simulink model "update"  (R2024a)
settings: Solver=VariableStepAuto  StartTime=0.0  StopTime=10.0  RelTol=1e-3
values from neighbouring files (symbols this model uses):
  c = 0.004    [model_constants.m]
  g = 9.81    [model_constants.m]
  J = 10.183e-4    (= 0.0010183)    [model_constants.m]
  k = 0.1    [model_constants.m]
  ke = 0.083    [model_constants.m]
  ki = 0.004    [model_constants.m]
  L = 0.134    [model_constants.m]
  m = 43.4    [model_constants.m]
  R = 0.5    [model_constants.m]
  x = 2    [model_constants.m]
libraries: simulink x2
settings Model: PacingRate=0.280000  Creator=tinas  LastModifiedBy=tinas

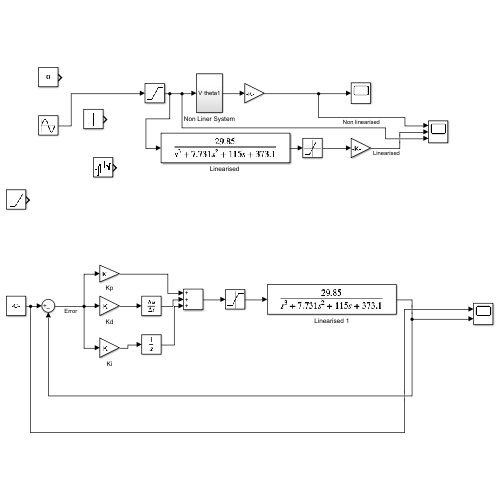
[thumbnail: Simulink's stored preview of the top-level diagram]
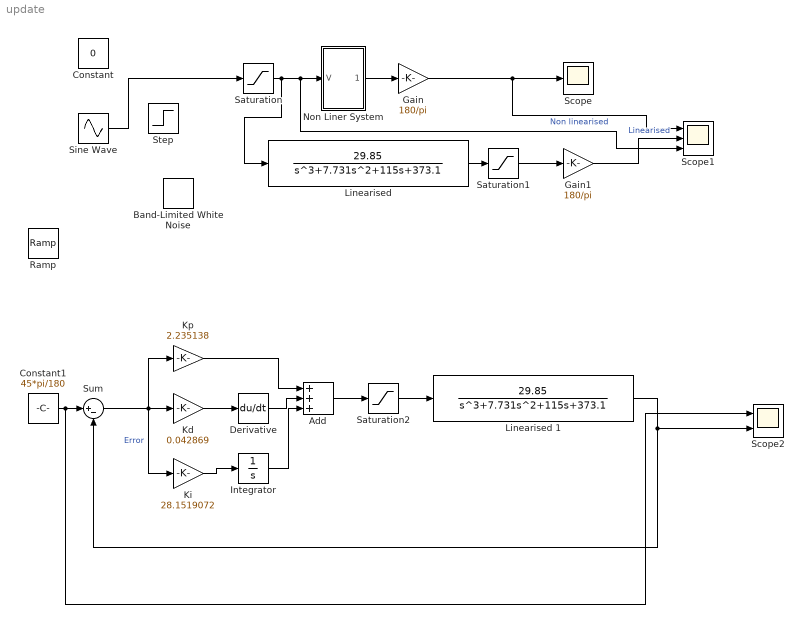
== system update ==
  Add : Sum  Inputs=+++
  Band-Limited White Noise : simulink/Sources/Band-Limited White Noise  Cov=[0.1]  Ts=0.1  seed=[23341]
  Constant : Constant  Value=0
  Constant1 : Constant  Value=45*pi/180
  Derivative : Derivative
  Gain : Gain  Gain=180/pi
  Gain1 : Gain  Gain=180/pi
  Integrator : Integrator
  Kd : Gain  Gain=0.042869
  Ki : Gain  Gain=28.1519072
  Kp : Gain  Gain=2.235138
  "Linearised " : TransferFcn  Numerator=[29.85]  Denominator="[1 7.731  115  373.1]"
  Linearised 1 : TransferFcn  Numerator=[29.85]  Denominator="[1 7.731  115  373.1]"
  Non Liner System : Subsystem
  Ramp : simulink/Sources/Ramp  slope=1  start=0  InitialOutput=0
  Saturation : Saturate  UpperLimit=20  LowerLimit=-20
  Saturation1 : Saturate  UpperLimit=pi/2  LowerLimit=-pi/2
  Saturation2 : Saturate  UpperLimit=100000000000000  LowerLimit=-100000000000000000000
  Scope : Scope
  Scope1 : Scope  NumInputPorts=3
  Scope2 : Scope  NumInputPorts=2
  Sine Wave : Sin  SampleTime=0
  Step : Step  SampleTime=0
  Sum : Sum  Inputs=|+-
  wires:
  Gain/1 -> Scope1/1, Scope/1  "Non linearised"
  Sine Wave/1 -> Saturation/1
  Saturation/1 -> "Linearised "/1, Scope1/3, Non Liner System/1(V)
  Non Liner System/1(theta1) -> Gain/1
  Gain1/1 -> Scope1/2  "Linearised"
  "Linearised "/1 -> Saturation1/1
  Saturation1/1 -> Gain1/1
  Saturation2/1 -> Linearised 1/1
  Add/1 -> Saturation2/1
  Kp/1 -> Add/1
  Kd/1 -> Derivative/1
  Derivative/1 -> Add/2
  Ki/1 -> Integrator/1
  Integrator/1 -> Add/3
  Sum/1 -> Ki/1, Kp/1, Kd/1  "Error"
  Constant1/1 -> Scope2/1, Sum/1
  Linearised 1/1 -> Scope2/2, Sum/2

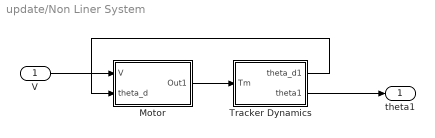
== system update/Non Liner System ==
  V : Inport
  Motor : Subsystem
  Tracker Dynamics : Subsystem
  theta1 : Outport
  wires:
  Motor/1(Out1) -> Tracker Dynamics/1(Tm)
  Tracker Dynamics/1(theta_d1) -> Motor/2(theta_d)
  V/1 -> Motor/1(V)
  Tracker Dynamics/2(theta1) -> theta1/1

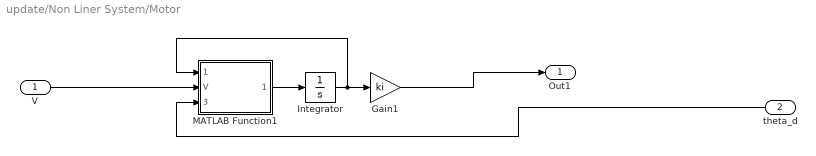
== system update/Non Liner System/Motor ==
  V : Inport
  theta_d : Inport  Port=2
  Gain1 : Gain  Gain=ki
  Integrator : Integrator
  MATLAB Function1 : MATLAB Function  TreatAsAtomicUnit=on
  Out1 : Outport
  wires:
  Integrator/1 -> MATLAB Function1/1(current), Gain1/1
  Gain1/1 -> Out1/1
  MATLAB Function1/1(current_dot) -> Integrator/1
  V/1 -> MATLAB Function1/2(V)
  theta_d/1 -> MATLAB Function1/3(theta_d)

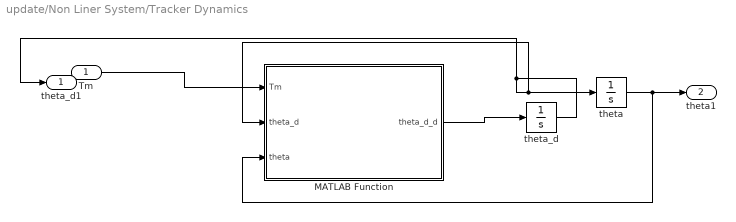
== system update/Non Liner System/Tracker Dynamics ==
  Tm : Inport
  MATLAB Function : MATLAB Function  TreatAsAtomicUnit=on
  theta : Integrator  LimitOutput=on  UpperSaturationLimit=pi/2  LowerSaturationLimit=-pi/2
  theta_d : Integrator
  theta_d1 : Outport
  theta1 : Outport  Port=2
  wires:
  theta_d/1 -> theta_d1/1, theta/1, MATLAB Function/2(theta_d)
  Tm/1 -> MATLAB Function/1(Tm)
  MATLAB Function/1(theta_d_d) -> theta_d/1
  theta/1 -> theta1/1, MATLAB Function/3(theta)

== matlab function update/Non Liner System/Motor/MATLAB Function1 ==
  data: current input; current_dot output; V input; theta_d input; ke parameter; L parameter; R parameter
function current_dot = fcn(current,V,theta_d,ke, L, R)



current_dot=(V-ke*theta_d-R*current)/L;

end

== matlab function update/Non Liner System/Tracker Dynamics/MATLAB Function ==
  data: Tm input; theta_d_d output; theta_d input; theta input; c parameter; k parameter; J parameter; m parameter; g parameter; x parameter
function theta_d_d = fcn(Tm,theta_d,theta,c, k, J,m, g,x)

theta_d_d=(Tm-c*theta_d-k*theta-x*m*g*cos(theta))/J;
end
